simulink model "mic_input_2d"  (R2013b)
settings: Solver=ode45  StartTime=0.0  StopTime=.01  RelTol=1e-3
libraries: dspsrcs4 x4
settings Model: Creator=nryan1_guest  LastModifiedBy=nryan1_guest

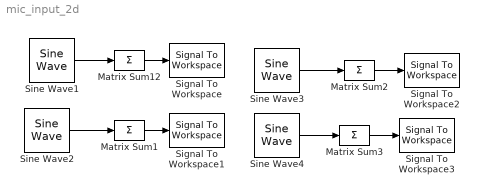
== system mic_input_2d ==
  Matrix Sum{1..3,12} (4 alike) : Sum  Inputs=+  CollapseMode=Specified dimension  CollapseDim=2  SampleTime=1/44100
  Signal To Workspace : SignalToWorkspace  VariableName=mic1
      settings: CopyFcn=dspblkcopystw(gcbh);
  Signal To Workspace1 : SignalToWorkspace  VariableName=mic2
      settings: CopyFcn=dspblkcopystw(gcbh);
  Signal To Workspace2 : SignalToWorkspace  VariableName=mic3
      settings: CopyFcn=dspblkcopystw(gcbh);
  Signal To Workspace3 : SignalToWorkspace  VariableName=mic4
      settings: CopyFcn=dspblkcopystw(gcbh);
  Sine Wave{1..4} (4 alike) : dspsrcs4/Sine Wave  Amplitude=5  Frequency=1000  Phase=0  SampleMode=Discrete  OutComplex=Real  CompMethod=Trigonometric fcn  TableSize=Speed  SampleTime=1/44100  SamplesPerFrame=1  ResetState=Restart at time zero  dataType=double  wordLen=16  udDataType=sfix(16)  fracBitsMode=Best precision  numFracBits=15  OutDataTypeStr=double  LastOutDataTypeStr=double
  wires:
  Sine Wave1/1 -> Matrix Sum12/1
  Matrix Sum12/1 -> Signal To Workspace/1
  Sine Wave2/1 -> Matrix Sum1/1
  Matrix Sum1/1 -> Signal To Workspace1/1
  Sine Wave3/1 -> Matrix Sum2/1
  Matrix Sum2/1 -> Signal To Workspace2/1
  Sine Wave4/1 -> Matrix Sum3/1
  Matrix Sum3/1 -> Signal To Workspace3/1
